simulink model "sliding_car"  (R2017a)
settings: Solver=VariableStepAuto  StartTime=0.0  StopTime=tf  RelTol=1e-3
values from neighbouring files (symbols this model uses):
  a = double(perc*D)    [init_vars.m]
  Cp_1 = 0    [init_vars.m]
  Cp_2 = 0    [init_vars.m]
  Fz_1 = g*(mc/4 + mi)    [init_vars.m]
  Fz_2 = g*(mc/4 + mi)    [init_vars.m]
  mu_1 = 1e-3    (= 0.001)    [init_vars.m]
  mu_2 = 1e-3    (= 0.001)    [init_vars.m]
  x0 = double(subs([qs; ps], [sys.descrip.syms.'; delta_i],                   [sys.descrip.model_params.'; delta_i_num]))    [init_vars.m]    (also in sim_blockdiagram.m)
undefined symbols (not defined in the file or in its folder): g, Ic_33, Ii_11, Ii_21, Ii_22, Ii_31, Ii_32, Ii_33, Il_11, Il_21, Il_22, Il_31, Il_32, Il_33, Io_11, Io_21, Io_22, Io_31, Io_32, Io_33, Ir_11, Ir_21, Ir_22, Ir_31, Ir_32, Ir_33, L, Lc, mc, mi, ml, mo, mr, R, sys, w
(part 5 of 5)

== matlab function sliding_car/Vehicle/Steering automobile model/Mass block/H ==
  data: C_1delta input; H output; M input
function H = ConstrinedMassMatrix(C_1delta, M)
% MASSMATRIX
%    This function was generated by the Symbolic Math Toolbox version 7.2.
%    16-Oct-2020 11:55:07

    H = C_1delta'*M*C_1delta;
end

== matlab function sliding_car/Vehicle/Sliding coefficients ==
  data: t input; kappa_1 output; kappa_2 output; alpha_1 output; alpha_2 output; dkappa_1 output; dkappa_2 output; dalpha_1 output; dalpha_2 output
function [kappa_1, kappa_2, alpha_1, alpha_2, ...
          dkappa_1, dkappa_2, dalpha_1, dalpha_2] = friction_force(t)
%     kappa_1 = -0.5;
%     kappa_2 = -0.5;
%     alpha_1 = 10*pi/180;
%     alpha_2 = 10*pi/180;

    kappa_1 = 0;
    kappa_2 = 0;
    alpha_1 = 0;
    alpha_2 = 0;


    dkappa_1 = 0;
    dkappa_2 = 0;
    dalpha_1 = 0;
    dalpha_2 = 0;
end

== matlab function sliding_car/Vehicle/Steering automobile model/Mass block/inv H ==
  data: matrix input; inv_matrix output
function inv_matrix = matrix_inverse(matrix)
% MASSMATRIX
%    This function was generated by the Symbolic Math Toolbox version 7.2.
%    16-Oct-2020 11:55:07

    inv_matrix = inv(matrix);
end

== matlab function sliding_car/Vehicle/Steering automobile model/Mass block/inverse M ==
  data: matrix input; inv_matrix output
function inv_matrix = matrix_inverse(matrix)
% MASSMATRIX
%    This function was generated by the Symbolic Math Toolbox version 7.2.
%    16-Oct-2020 11:55:07

    inv_matrix = inv(matrix);
end

== matlab function sliding_car/Vehicle/Steering automobile model/Mass block/square root M ==
  data: matrix input; square_root_matrix output
function square_root_matrix = matrix_square_root(matrix)
% MASSMATRIX
%    This function was generated by the Symbolic Math Toolbox version 7.2.
%    16-Oct-2020 11:55:07

    square_root_matrix = real(sqrtm(matrix));
end

== matlab function sliding_car/Vehicle/Steering automobile model/Mass block/inverse M1 ==
  data: matrix input; inv_matrix output
function inv_matrix = matrix_inverse(matrix)
% MASSMATRIX
%    This function was generated by the Symbolic Math Toolbox version 7.2.
%    16-Oct-2020 11:55:07

    inv_matrix = inv(matrix);
end

== matlab function sliding_car/Vehicle/Steering automobile model/Auxiliary matrices/qp ==
  data: x input; kappa_1 input; kappa_2 input; alpha_1 input; alpha_2 input; Ii_11 parameter; Ii_21 parameter; Ii_22 parameter; Ii_31 parameter; Ii_32 parameter; Ii_33 parameter; Il_11 parameter; Il_21 parameter; Il_22 parameter; Il_31 parameter; Il_32 parameter; Il_33 parameter; Io_11 parameter; Io_21 parameter; Io_22 parameter; Io_31 parameter; Io_32 parameter; Io_33 parameter; Ir_11 parameter; Ir_21 parameter; Ir_22 parameter; Ir_31 parameter; Ir_32 parameter; Ir_33 parameter; Lc parameter; mc parameter; mi parameter; ml parameter; mo parameter; mr parameter; L parameter; w parameter; qp output
function qp = KinematicVector(x, kappa_1, kappa_2, alpha_1, alpha_2, ...
                              Ii_11, Ii_21, Ii_22, Ii_31, Ii_32, Ii_33, ...
                              Il_11, Il_21, Il_22, Il_31, Il_32, Il_33, ...
                              Io_11, Io_21, Io_22, Io_31, Io_32, Io_33, ...
                              Ir_11, Ir_21, Ir_22, Ir_31, Ir_32, Ir_33, ...
                              Lc, mc, mi, ml, mo, mr, L, w)
% INPUTMATRIX
%    Q = INPUTMATRIX(II_11,II_21,II_22,II_31,II_32,II_33,IL_11,IL_21,IL_22,IL_31,IL_32,IL_33,IO_11,IO_21,IO_22,IO_31,IO_32,IO_33,IR_11,IR_21,IR_22,IR_31,IR_32,IR_33,L,LC,DELTA_I,DELTA_O,DELTAP_I,DELTAP_O,F_PHI_I,F_PHI_L,F_PHI_O,F_PHI_R,MC,MI,ML,MO,MR,PHI_I,PHI_L,PHI_O,PHI_R,PHIP_I,PHIP_L,PHIP_O,PHIP_R,THETAP,THETA,W)

%    This function was generated by the Symbolic Math Toolbox version 7.2.
%    16-Oct-2020 13:53:49

    x_pos =  x(1);
    y_pos =  x(2);
    theta =  x(3);

    delta_i = x(4);
    delta_o = x(5);

    phi_i = x(6);
    phi_l = x(7);
    phi_o = x(8);
    phi_r = x(9);
    
    p1 = x(10);
    p2 = x(11);
    p3 = x(12);
    
    % C_1delta*p
    t2 = delta_i+theta;
    t3 = cos(t2);
    t4 = tan(delta_i);
    t5 = t4+3.0;
    t6 = 1.0./t5;
    t7 = t4.*t6.*3.0;
    t8 = atan(t7);
    t9 = t8+theta;
    t10 = cos(t9);
    t11 = 1.0./t5.^2;
    t12 = t4.*6.0;
    t13 = t4.^2;
    t14 = t13.*1.0e1;
    t15 = t12+t14+9.0;
    t16 = t11.*t15;
    t17 = sqrt(t16);
    t18 = sin(t2);
    t19 = tan(alpha_1);
    t20 = cos(delta_i);
    t21 = sin(delta_i);
    t22 = tan(alpha_2);
    t23 = delta_o+theta;
    t24 = sin(t23);
    t25 = cos(delta_o);
    t26 = sin(delta_o);
    t27 = sin(t9);
    t28 = t10.^2;
    t29 = t27.^2;
    t30 = cos(t23);
    t31 = t3.*t10.*3.0;
    t32 = t3.*t27.*1.8e1;
    t33 = t18.*t27.*3.0;
    t34 = t3.*t4.*t27.*9.0;
    t35 = t17.*t20.*t28.*3.0;
    t36 = t17.*t21.*t28.*1.8e1;
    t37 = t17.*t20.*t29.*3.0;
    t38 = t17.*t21.*t29.*1.8e1;
    t39 = t4.*t17.*t20.*t28;
    t40 = t4.*t17.*t21.*t28.*6.0;
    t41 = t4.*t17.*t20.*t29;
    t42 = t4.*t17.*t21.*t29.*6.0;
    t43 = kappa_1.*t3.*t10.*t19.*1.8e1;
    t44 = kappa_1.*t10.*t18.*t19.*3.0;
    t45 = kappa_1.*t18.*t19.*t27.*1.8e1;
    t46 = kappa_1.*t3.*t4.*t10.*t19.*9.0;
    t47 = kappa_1.*t3.*t4.*t19.*t27.*1.7e1;
    t48 = kappa_1.*t4.*t18.*t19.*t27.*9.0;
    t49 = kappa_1.*t17.*t19.*t21.*t28.*3.0;
    t50 = kappa_1.*t17.*t19.*t21.*t29.*3.0;
    t51 = kappa_2.*t3.*t10.*t17.*t22.*t26.*3.0;
    t52 = kappa_2.*t10.*t17.*t21.*t22.*t30.*1.8e1;
    t53 = kappa_2.*t10.*t17.*t20.*t22.*t24.*3.0;
    t54 = kappa_2.*t3.*t17.*t22.*t25.*t27.*1.8e1;
    t55 = kappa_2.*t10.*t17.*t21.*t22.*t24.*1.8e1;
    t56 = kappa_2.*t3.*t17.*t22.*t26.*t27.*3.0;
    t57 = kappa_2.*t17.*t18.*t22.*t25.*t27.*1.8e1;
    t58 = kappa_2.*t17.*t20.*t22.*t24.*t27.*3.0;
    t59 = kappa_2.*t17.*t18.*t22.*t26.*t27.*3.0;
    t60 = kappa_2.*t17.*t21.*t22.*t24.*t27.*1.8e1;
    t61 = kappa_1.*kappa_2.*t3.*t19.*t22.*t24.*1.5e1;
    t62 = kappa_1.*t4.*t17.*t19.*t21.*t28;
    t63 = kappa_1.*t4.*t17.*t19.*t21.*t29;
    t64 = kappa_2.*t3.*t10.*t17.*t22.*t25.*1.8e1;
    t65 = kappa_2.*t10.*t17.*t20.*t22.*t30.*3.0;
    t66 = kappa_1.*kappa_2.*t3.*t4.*t19.*t22.*t24.*2.6e1;
    t67 = kappa_2.*t3.*t4.*t10.*t17.*t22.*t25.*6.0;
    t68 = kappa_2.*t4.*t10.*t17.*t20.*t22.*t30;
    t69 = kappa_2.*t3.*t4.*t10.*t17.*t22.*t26;
    t70 = kappa_2.*t4.*t10.*t17.*t21.*t22.*t30.*6.0;
    t71 = kappa_2.*t4.*t10.*t17.*t20.*t22.*t24;
    t72 = kappa_2.*t3.*t4.*t17.*t22.*t25.*t27.*6.0;
    t73 = kappa_2.*t4.*t10.*t17.*t21.*t22.*t24.*6.0;
    t74 = kappa_2.*t3.*t4.*t17.*t22.*t26.*t27;
    t75 = kappa_2.*t4.*t17.*t18.*t22.*t25.*t27.*6.0;
    t76 = kappa_2.*t4.*t17.*t20.*t22.*t24.*t27;
    t77 = kappa_2.*t4.*t17.*t18.*t22.*t26.*t27;
    t78 = kappa_2.*t4.*t17.*t21.*t22.*t24.*t27.*6.0;
    t79 = kappa_1.*kappa_2.*t3.*t10.*t17.*t19.*t22.*t25.*1.8e1;
    t80 = kappa_1.*kappa_2.*t3.*t10.*t17.*t19.*t22.*t26.*3.0;
    t81 = kappa_1.*kappa_2.*t10.*t17.*t19.*t21.*t22.*t30.*3.0;
    t82 = kappa_1.*kappa_2.*t10.*t17.*t18.*t19.*t22.*t25.*1.8e1;
    t83 = kappa_1.*kappa_2.*t17.*t19.*t20.*t22.*t27.*t30.*1.8e1;
    t84 = kappa_1.*kappa_2.*t10.*t17.*t18.*t19.*t22.*t26.*3.0;
    t85 = kappa_1.*kappa_2.*t10.*t17.*t19.*t21.*t22.*t24.*3.0;
    t86 = kappa_1.*kappa_2.*t17.*t18.*t19.*t22.*t25.*t27.*1.8e1;
    t87 = kappa_1.*kappa_2.*t17.*t18.*t19.*t22.*t26.*t27.*3.0;
    t88 = kappa_1.*kappa_2.*t17.*t19.*t21.*t22.*t24.*t27.*3.0;
    t89 = kappa_1.*kappa_2.*t3.*t4.*t10.*t17.*t19.*t22.*t25.*6.0;
    t90 = kappa_1.*kappa_2.*t3.*t4.*t10.*t17.*t19.*t22.*t26;
    t91 = kappa_1.*kappa_2.*t4.*t10.*t17.*t19.*t21.*t22.*t30;
    t92 = kappa_1.*kappa_2.*t4.*t10.*t17.*t18.*t19.*t22.*t25.*6.0;
    t93 = kappa_1.*kappa_2.*t4.*t17.*t19.*t20.*t22.*t27.*t30.*6.0;
    t94 = kappa_1.*kappa_2.*t4.*t10.*t17.*t18.*t19.*t22.*t26;
    t95 = kappa_1.*kappa_2.*t4.*t10.*t17.*t19.*t21.*t22.*t24;
    t96 = kappa_1.*kappa_2.*t4.*t17.*t18.*t19.*t22.*t25.*t27.*6.0;
    t97 = kappa_1.*kappa_2.*t4.*t17.*t18.*t19.*t22.*t26.*t27;
    t98 = kappa_1.*kappa_2.*t4.*t17.*t19.*t21.*t22.*t24.*t27;
    t101 = t10.*t18.*1.8e1;
    t102 = t3.*t4.*t10.*1.7e1;
    t103 = t4.*t10.*t18.*9.0;
    t104 = t4.*t18.*t27.*1.7e1;
    t105 = kappa_1.*t3.*t19.*t27.*3.0;
    t106 = kappa_2.*t3.*t22.*t30.*1.5e1;
    t107 = kappa_2.*t18.*t22.*t24.*1.5e1;
    t108 = kappa_1.*t4.*t10.*t18.*t19.*1.7e1;
    t109 = kappa_2.*t3.*t4.*t22.*t30.*2.6e1;
    t110 = kappa_1.*t17.*t19.*t20.*t28.*1.8e1;
    t111 = kappa_1.*t17.*t19.*t20.*t29.*1.8e1;
    t112 = kappa_2.*t4.*t18.*t22.*t24.*2.6e1;
    t113 = kappa_2.*t10.*t17.*t18.*t22.*t25.*1.8e1;
    t114 = kappa_2.*t17.*t20.*t22.*t27.*t30.*3.0;
    t115 = kappa_2.*t10.*t17.*t18.*t22.*t26.*3.0;
    t116 = kappa_2.*t17.*t21.*t22.*t27.*t30.*1.8e1;
    t117 = kappa_1.*kappa_2.*t18.*t19.*t22.*t30.*1.5e1;
    t118 = kappa_1.*t4.*t17.*t19.*t20.*t28.*6.0;
    t119 = kappa_1.*t4.*t17.*t19.*t20.*t29.*6.0;
    t120 = kappa_1.*kappa_2.*t4.*t18.*t19.*t22.*t30.*2.6e1;
    t121 = kappa_2.*t4.*t10.*t17.*t18.*t22.*t25.*6.0;
    t122 = kappa_2.*t4.*t17.*t20.*t22.*t27.*t30;
    t123 = kappa_2.*t4.*t10.*t17.*t18.*t22.*t26;
    t124 = kappa_2.*t4.*t17.*t21.*t22.*t27.*t30.*6.0;
    t125 = kappa_1.*kappa_2.*t10.*t17.*t19.*t20.*t22.*t30.*1.8e1;
    t126 = kappa_1.*kappa_2.*t10.*t17.*t19.*t20.*t22.*t24.*1.8e1;
    t127 = kappa_1.*kappa_2.*t3.*t17.*t19.*t22.*t25.*t27.*1.8e1;
    t128 = kappa_1.*kappa_2.*t3.*t17.*t19.*t22.*t26.*t27.*3.0;
    t129 = kappa_1.*kappa_2.*t17.*t19.*t21.*t22.*t27.*t30.*3.0;
    t130 = kappa_1.*kappa_2.*t17.*t19.*t20.*t22.*t24.*t27.*1.8e1;
    t131 = kappa_1.*kappa_2.*t4.*t10.*t17.*t19.*t20.*t22.*t30.*6.0;
    t132 = kappa_1.*kappa_2.*t4.*t10.*t17.*t19.*t20.*t22.*t24.*6.0;
    t133 = kappa_1.*kappa_2.*t3.*t4.*t17.*t19.*t22.*t25.*t27.*6.0;
    t134 = kappa_1.*kappa_2.*t3.*t4.*t17.*t19.*t22.*t26.*t27;
    t135 = kappa_1.*kappa_2.*t4.*t17.*t19.*t21.*t22.*t27.*t30;
    t136 = kappa_1.*kappa_2.*t4.*t17.*t19.*t20.*t22.*t24.*t27.*6.0;
    t99 = t31+t32+t33+t34+t35+t36+t37+t38+t39+t40+t41+t42+t43+t44+...
          t45+t46+t47+t48+t49+t50+t51+t52+t53+t54+t55+t56+t57+t58+...
          t59+t60+t61+t62+t63+t64+t65+t66+t67+t68+t69+t70+t71+t72+...
          t73+t74+t75+t76+t77+t78+t79+t80+t81+t82+t83+t84+t85+t86+...
          t87+t88+t89+t90+t91+t92+t93+t94+t95+t96+t97+t98-t101-t102-...
          t103-t104-t105-t106-t107-t108-t109-t110-t111-t112-t113-t114-...
          t115-t116-t117-t118-t119-t120-t121-t122-t123-t124-t125-t126-...
          t127-t128-t129-t130-t131-t132-t133-t134-t135-t136;
    t100 = 1.0./t99;
    t137 = t18.^2;
    t138 = t3.^2;
    
    qp = [p2.*t100.*(t3.*3.0-t3.*t4.*1.7e1+kappa_1.*t18.*t19.*3.0+t10.*t17.*t20.*3.0+t10.*t17.*t21.*1.8e1-kappa_1.*t4.*t18.*t19.*1.7e1+t4.*t10.*t17.*t20+t4.*t10.*t17.*t21.*6.0-kappa_1.*t10.*t17.*t19.*t20.*1.8e1+kappa_1.*t10.*t17.*t19.*t21.*3.0+kappa_2.*t3.*t17.*t22.*t25.*1.8e1+kappa_2.*t3.*t17.*t22.*t26.*3.0+kappa_2.*t17.*t20.*t22.*t24.*3.0+kappa_2.*t17.*t21.*t22.*t24.*1.8e1-kappa_1.*t4.*t10.*t17.*t19.*t20.*6.0+kappa_1.*t4.*t10.*t17.*t19.*t21+kappa_2.*t3.*t4.*t17.*t22.*t25.*6.0+kappa_2.*t3.*t4.*t17.*t22.*t26+kappa_2.*t4.*t17.*t20.*t22.*t24+kappa_2.*t4.*t17.*t21.*t22.*t24.*6.0+kappa_1.*kappa_2.*t17.*t18.*t19.*t22.*t25.*1.8e1+kappa_1.*kappa_2.*t17.*t18.*t19.*t22.*t26.*3.0-kappa_1.*kappa_2.*t17.*t19.*t20.*t22.*t24.*1.8e1+kappa_1.*kappa_2.*t17.*t19.*t21.*t22.*t24.*3.0+kappa_1.*kappa_2.*t4.*t17.*t18.*t19.*t22.*t25.*6.0+kappa_1.*kappa_2.*t4.*t17.*t18.*t19.*t22.*t26-kappa_1.*kappa_2.*t4.*t17.*t19.*t20.*t22.*t24.*6.0+kappa_1.*kappa_2.*t4.*t17.*t19.*t21.*t22.*t24).*3.442462000000001e-1;
          p2.*t100.*(t18.*3.0-t4.*t18.*1.7e1-kappa_1.*t3.*t19.*3.0+t17.*t20.*t27.*3.0+t17.*t21.*t27.*1.8e1+kappa_1.*t3.*t4.*t19.*1.7e1+t4.*t17.*t20.*t27+t4.*t17.*t21.*t27.*6.0-kappa_1.*t17.*t19.*t20.*t27.*1.8e1+kappa_2.*t17.*t18.*t22.*t25.*1.8e1+kappa_1.*t17.*t19.*t21.*t27.*3.0+kappa_2.*t17.*t18.*t22.*t26.*3.0-kappa_2.*t17.*t20.*t22.*t30.*3.0-kappa_2.*t17.*t21.*t22.*t30.*1.8e1-kappa_1.*t4.*t17.*t19.*t20.*t27.*6.0+kappa_2.*t4.*t17.*t18.*t22.*t25.*6.0+kappa_1.*t4.*t17.*t19.*t21.*t27+kappa_2.*t4.*t17.*t18.*t22.*t26-kappa_2.*t4.*t17.*t20.*t22.*t30-kappa_2.*t4.*t17.*t21.*t22.*t30.*6.0-kappa_1.*kappa_2.*t3.*t17.*t19.*t22.*t25.*1.8e1-kappa_1.*kappa_2.*t3.*t17.*t19.*t22.*t26.*3.0+kappa_1.*kappa_2.*t17.*t19.*t20.*t22.*t30.*1.8e1-kappa_1.*kappa_2.*t17.*t19.*t21.*t22.*t30.*3.0-kappa_1.*kappa_2.*t3.*t4.*t17.*t19.*t22.*t25.*6.0-kappa_1.*kappa_2.*t3.*t4.*t17.*t19.*t22.*t26+kappa_1.*kappa_2.*t4.*t17.*t19.*t20.*t22.*t30.*6.0-kappa_1.*kappa_2.*t4.*t17.*t19.*t21.*t22.*t30).*3.442462000000001e-1;
          p2.*t5.*t17.*t100.*(t10.*t18-t3.*t27-kappa_1.*t3.*t10.*t19+kappa_2.*t3.*t22.*t30-kappa_1.*t18.*t19.*t27+kappa_2.*t18.*t22.*t24-kappa_1.*kappa_2.*t3.*t19.*t22.*t24+kappa_1.*kappa_2.*t18.*t19.*t22.*t30).*4.589949333333334e-1;
          (p1.*t15.*(1.0./9.0))./(t13+1.0);
          p1;
          p2.*t100.*(kappa_1.*t19+1.0).*(t137.*3.0+t138.*3.0-t4.*t137.*1.7e1-t4.*t138.*1.7e1+t3.*t10.*t17.*t20.*3.0+t3.*t10.*t17.*t21.*1.8e1-t10.*t17.*t18.*t20.*1.8e1+t10.*t17.*t18.*t21.*3.0+t3.*t17.*t20.*t27.*1.8e1-t3.*t17.*t21.*t27.*3.0+t17.*t18.*t20.*t27.*3.0+t17.*t18.*t21.*t27.*1.8e1+kappa_2.*t17.*t22.*t25.*t137.*1.8e1+kappa_2.*t17.*t22.*t25.*t138.*1.8e1+kappa_2.*t17.*t22.*t26.*t137.*3.0+kappa_2.*t17.*t22.*t26.*t138.*3.0+t3.*t4.*t10.*t17.*t20+t3.*t4.*t10.*t17.*t21.*6.0-t4.*t10.*t17.*t18.*t20.*6.0+t4.*t10.*t17.*t18.*t21+t3.*t4.*t17.*t20.*t27.*6.0-t3.*t4.*t17.*t21.*t27+t4.*t17.*t18.*t20.*t27+t4.*t17.*t18.*t21.*t27.*6.0+kappa_2.*t3.*t17.*t20.*t22.*t24.*3.0+kappa_2.*t3.*t17.*t21.*t22.*t24.*1.8e1-kappa_2.*t3.*t17.*t20.*t22.*t30.*1.8e1+kappa_2.*t3.*t17.*t21.*t22.*t30.*3.0-kappa_2.*t17.*t18.*t20.*t22.*t24.*1.8e1+kappa_2.*t17.*t18.*t21.*t22.*t24.*3.0-kappa_2.*t17.*t18.*t20.*t22.*t30.*3.0-kappa_2.*t17.*t18.*t21.*t22.*t30.*1.8e1+kappa_2.*t4.*t17.*t22.*t25.*t137.*6.0+kappa_2.*t4.*t17.*t22.*t25.*t138.*6.0+kappa_2.*t4.*t17.*t22.*t26.*t137+kappa_2.*t4.*t17.*t22.*t26.*t138+kappa_2.*t3.*t4.*t17.*t20.*t22.*t24+kappa_2.*t3.*t4.*t17.*t21.*t22.*t24.*6.0-kappa_2.*t3.*t4.*t17.*t20.*t22.*t30.*6.0+kappa_2.*t3.*t4.*t17.*t21.*t22.*t30-kappa_2.*t4.*t17.*t18.*t20.*t22.*t24.*6.0+kappa_2.*t4.*t17.*t18.*t21.*t22.*t24-kappa_2.*t4.*t17.*t18.*t20.*t22.*t30-kappa_2.*t4.*t17.*t18.*t21.*t22.*t30.*6.0);
          p2;
          p3.*t6.*3.0;
          p3];

== matlab function sliding_car/Vehicle/Steering automobile model/Friction model ==
  data: q input; p input; kappa_1 input; kappa_2 input; alpha_1 input; alpha_2 input; C_1delta input; mc parameter; mi parameter; C_fric output; g parameter; a parameter; Cp_1 parameter; mu_1 parameter; Fz_1 parameter; Cp_2 parameter; mu_2 parameter; Fz_2 parameter
function C_fric = friction_force(q, p, kappa_1, kappa_2, alpha_1, alpha_2, C_1delta, ...
                                 mc, mi, g, a, Cp_1, mu_1, Fz_1, Cp_2, mu_2, Fz_2)
    
    delta_i = q(4);
    delta_o = q(5);
    theta = q(3);
    
    w_delta_o = p(1);
    w_phi_o = p(2);
    w_phi_l = p(3);
    
    qp = C_1delta*p;
    
    w_theta = qp(3);
    w_delta_i = qp(4);
    w_phi_i = qp(6);
    w_phi_r = qp(end-1);

    R_th_i = rot2d(theta + delta_i);
    R_th_o = rot2d(theta + delta_o);
    R_th = rot2d(theta);
    
    n = length(q);
    
    % Canonical vectors
    e_th = canon_Rn(n, 3);
    e_compl = zeros(n-2, 1);
    
    n = length(q);
    Iq_3 = eye(n-2);
    
    R6_th_i = blkdiag(R_th_i, Iq_3);
    R6_th_o = blkdiag(R_th_o, Iq_3);
    R6_th = blkdiag(R_th, Iq_3);
    
    sigma_x_1 = kappa_1/(kappa_1 + 1);
    sigma_y_1 = tan(alpha_1)/(kappa_1 + 1);
    
    sigma_x_2 = kappa_2/(kappa_2 + 1);
    sigma_y_2 = tan(alpha_2)/(kappa_2 + 1);
    
    sigma_1 = terop((sigma_x_1 == 0)||(sigma_y_1 == 0), ...
                    sqrt(sigma_x_1^2 + sigma_y_1^2), 1);
    sigma_2 = terop((sigma_x_2 == 0)||(sigma_y_2 == 0), ...
                     sqrt(sigma_x_2^2 + sigma_y_2^2), 1);
                 
    theta_1 = double((2/3)*(Cp_1*a^2/(mu_1*Fz_1)));
    theta_2 = double((2/3)*(Cp_2*a^2/(mu_2*Fz_2)));
    
    lambda_1 = 1 - theta_1*sigma_1;
    lambda_2 = 1 - theta_2*sigma_2;
    
    if(theta_1 ~= 0)
        sigma_sl_1 = 1/theta_1;
        Fz_1 = (mc/4 + mi)*g;
        
        if(sigma_1 <= sigma_sl_1)
            F_1 = mu_1*Fz_1*(1 - lambda_1^3);
        else
            F_1 = mu_1*Fz_1;
        end
        
        F1_vec = F_1*[sigma_x_1; sigma_y_1]/sigma_1;
        t_lambda_1 = (lambda_1^3/(1 + lambda_1 + lambda_1^2))*a;
    
        Mz_1 = -t_lambda_1*F1_vec(2);
    else
        F1_vec = [0; 0];
        Mz_1 = 0;
    end
    
    if(theta_2 ~= 0)
        sigma_sl_2 = 1/theta_2; 
        Fz_2 = (mc/4 + mi)*g;

        if(sigma_2 <= sigma_sl_2)
            F_2 = mu_2*Fz_2*(1 - lambda_2^3);
        else
            F_2 = mu_2*Fz_2;
        end

        F2_vec = F_2*[sigma_x_2; sigma_y_2]/sigma_2;
        t_lambda_2 = (lambda_2^3/(1 + lambda_2 + lambda_2^2))*a;
        Mz_2 = -t_lambda_2*F2_vec(2);
    else
        F2_vec = [0; 0];
        Mz_2 = 0;
    end
    
    C_i = -R6_th_i*[F1_vec; e_compl] + e_th*Mz_1;
    C_o = -R6_th_o*[F2_vec; e_compl] + e_th*Mz_2;
    
    C_fric = C_i + C_o;
end
